simulink model "mod_3_fichier_SI"  (R2019b)
settings: Solver=ode5  StartTime=0  StopTime=100  FixedStep=0.001  MaxStep=0.01  RelTol=1e-3  AbsTol=1e-3
values from neighbouring files (symbols this model uses):
  a = m/(M+m)    (= 0.0874524714829)    [cipendco.m]
  fc = 7.96    [cipendco.m]
  g = 9.81    [cipendco.m]
  J = 0.099    [cipendco.m]
  k0_x1 = K(1)    [cipendco.m]
  k0_x3 = K(3)    [cipendco.m]
  k1_x1 = K(2)    [cipendco.m]
  k1_x3 = K(4)    [cipendco.m]
  l = 0.36    [cipendco.m]
  m = 0.23    [cipendco.m]
  M = 2.4    [cipendco.m]
settings Model: ExtModeTrigMode=oneshot  ExtModeArmWhenConnect=off  ExtModeAutoUpdateStatusClock=off  Creator=franckplestan  LastModifiedBy=15043
settings SolverCC: AutoScaleAbsTol=off
settings DataIOCC: SaveFormat=Array  SignalLoggingSaveFormat=ModelDataLogs  SaveOutput=off  ReturnWorkspaceOutputs=off  SignalLoggingName=sigsOut
settings OptimizationCC: BooleanDataType=off  ExpressionDepthLimit=2147483647  InitFltsAndDblsToZero=on  LifeSpan=inf
settings DebuggingCC: SaveWithParameterizedLinksMsg=none  UnderspecifiedInitializationDetection=Classic  MergeDetectMultiDrivingBlocksExec=none  SignalResolutionControl=TryResolveAllWithWarning  MultiTaskDSMMsg=warning  MultiTaskCondExecSysMsg=none  FcnCallInpInsideContextMsg=warning  StateNameClashWarn=warning  SFUnexpectedBacktrackingDiag=warning  SFNoUnconditionalDefaultTransitionDiag=warning  SFExecutionAtInitializationDiag=none  ArithmeticOperatorsInVariantConditions=warning
settings HardwareCC: ProdBitPerPointer=32  ProdBitPerSizeT=32  ProdBitPerPtrDiffT=32  ProdLargestAtomicFloat=None  ProdIntDivRoundTo=Undefined  ProdEndianess=Unspecified  ProdWordSize=32  ProdHWDeviceType=32-bit Generic  TargetUnknown=on
settings ModelReferenceCC: PropagateSignalLabelsOutOfModel=off
settings SFSimCC: CustomCodeUndefinedFunction=UseInterfaceOnly
settings CodeAppCC: StateflowObjectComments=on
settings GRTTargetCC: TargetLangStandard=C89/C90 (ANSI)  ModelReferenceCompliant=off  CompOptLevelCompliant=off  CombineOutputUpdateFcns=off  MatFileLogging=off  GRTInterface=on
settings ConfigComp: CovMetricSettings=dw  CovHtmlReporting=on  CovSaveCumulativeToWorkspaceVar=on  CovSaveSingleToWorkspaceVar=on

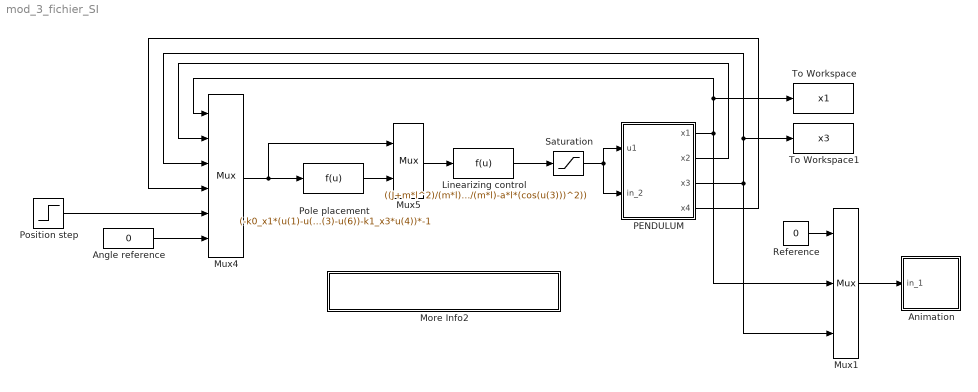
== system mod_3_fichier_SI ==
  Angle reference : Constant  Value=0
  Animation : Subsystem  mask(Pendulum plot){RefBlock=Reference}
      mask prompts: RefBlock "DC reference signal block name:"
      mask help: Pendulum plot
      mask Help: Pendulum animation function using Handle graphics.
      mask Display: plot([-10 10],[0 0],[-2 -2 2 2],[0 1 1 0],[0 3],[1 5])
  Linearizing control : Fcn  Expr=((J+m*l^2)/(m*l)-a*l*(cos(u(3)))^2)/(-a/m*cos(u(3)))*((u(7)+(a*l*sin(u(3))*cos(u(3))*u(4)^2)-g*sin(u(3))-a*fc/m*u(2)*cos(u(3)))/((J+m*l^2)/(m*l)-a*l*(cos(u(3)))^2))
  More Info2 : Subsystem
      settings: OpenFcn=cipendco_student
      mask Display: disp('Parameters initialization - File cipendco_student')
  Mux1 : Mux  Inputs=3
  Mux4 : Mux  Inputs=6
  Mux5 : Mux  Inputs=2
  PENDULUM : Subsystem
  Pole placement : Fcn  Expr=(-k0_x1*(u(1)-u(5))-k1_x1*u(2)-k0_x3*(u(3)-u(6))-k1_x3*u(4))*-1
  Position step : Step  Time=40  Before=-2  After=+2  SampleTime=0
  Reference : Constant  Value=0
  Saturation : Saturate  UpperLimit=24  LowerLimit=-24
  To Workspace : ToWorkspace  VariableName=x1  SampleTime=-1
  To Workspace1 : ToWorkspace  VariableName=x3  SampleTime=-1
  wires:
  Linearizing control/1 -> Saturation/1
  Angle reference/1 -> Mux4/6
  Pole placement/1 -> Mux5/2
  Mux4/1 -> Pole placement/1, Mux5/1
  Mux5/1 -> Linearizing control/1
  PENDULUM/4(x4) -> Mux4/4
  Saturation/1 -> PENDULUM/1(u1), PENDULUM/2(in_2)
  PENDULUM/1(x1) -> Mux4/1, To Workspace/1, Mux1/2
  PENDULUM/2(x2) -> Mux4/2
  PENDULUM/3(x3) -> Mux4/3, To Workspace1/1, Mux1/3
  Mux1/1 -> Animation/1(in_1)
  Reference/1 -> Mux1/1
  Position step/1 -> Mux4/5

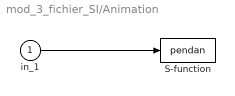
== system mod_3_fichier_SI/Animation ==
  in_1 : Inport
  S-function : S-Function  FunctionName=pendan  Parameters=RefBlock  SFunctionDeploymentMode=off  EnableBusSupport=off
      settings: DeleteFcn=pendan([],[],[],'DeleteBlock');
  wires:
  in_1/1 -> S-function/1

== system mod_3_fichier_SI/More Info2 ==

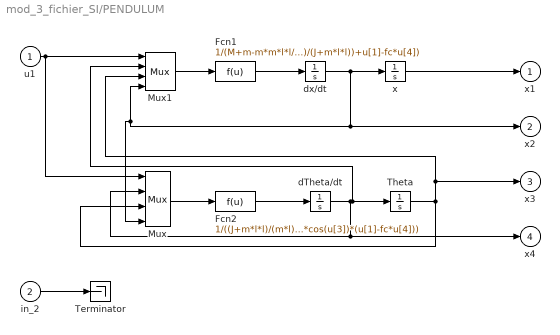
== system mod_3_fichier_SI/PENDULUM ==
  u1 : Inport
  in_2 : Inport  Port=2
  Fcn1 : Fcn  Expr=1/(M+m-m*m*l*l/(J+m*l*l)*power(cos(u[3]),2))*(m*sin(u[3])*(l*power(u[2],2)-m*l*l*g*cos(u[3])/(J+m*l*l))+u[1]-fc*u[4])
  Fcn2 : Fcn  Expr=1/((J+m*l*l)/(m*l)-a*l*power(cos(u[3]),2))*(-a*l*sin(u[3])*cos(u[3])*power(u[2],2)+g*sin(u[3])-a/m*cos(u[3])*(u[1]-fc*u[4]))
  Mux : Mux
  Mux1 : Mux
  Terminator : Terminator
  Theta : Integrator  InitialCondition=0.2
  dTheta/dt : Integrator
  dx/dt : Integrator
  x : Integrator  InitialCondition=0.5
  x1 : Outport  VectorParamsAs1DForOutWhenUnconnected=off
  x2 : Outport  Port=2  VectorParamsAs1DForOutWhenUnconnected=off
  x3 : Outport  Port=3  VectorParamsAs1DForOutWhenUnconnected=off
  x4 : Outport  Port=4  VectorParamsAs1DForOutWhenUnconnected=off
  wires:
  in_2/1 -> Terminator/1
  dx/dt/1 -> Mux/4, Mux1/4, x2/1, x/1
  x/1 -> x1/1
  Fcn2/1 -> dTheta/dt/1
  Mux/1 -> Fcn2/1
  Mux1/1 -> Fcn1/1
  Fcn1/1 -> dx/dt/1
  dTheta/dt/1 -> Theta/1, Mux1/2, Mux/2, x4/1
  u1/1 -> Mux/1, Mux1/1
  Theta/1 -> Mux1/3, x3/1, Mux/3
